simulink model "sldemo_househeatsolution"  (R2026a)
settings: Solver=ode45  StopTime=172800  FixedStep=1  AbsTol=1e-6
model workspace (MATLAB code in the model file):
  | % load initial conditions and physical properties from file
  | 
  | sldemo_househeat_data
undefined symbols (not defined in the file): c, cost, M, Mdot, Req, THeater, TinIC
libraries: simulink_extras x3
Description:
  | Thermal Model of a House
  | 
  | This demo illustrates how you can use Simulink(R) to create the thermal model of
  | a house. This system models the outdoor environment, the thermal
  | characteristics of the house, and the house heating system.
  | 
  | The sldemo_househeat_data.m file initializes data in the model workspace.
  | To make changes, you can edit the model workspace directly or edit the MATLAB(R) file
  | and re-load the model workspace.
  | 
  | To view the model workspace, select View > Model Explorer
  | from the Simulink editor.
  | 
  | Note: Time is given in units of hours
settings Model: ExtModeTrigMode=oneshot  ExtModeArmWhenConnect=off  ExtModeAutoUpdateStatusClock=off  Creator=The MathWorks, Inc.  LastModifiedBy=The MathWorks, Inc.
settings DataIOCC: ExternalInput=[]  InitialState=[]
settings OptimizationCC: BooleanDataType=off  InitFltsAndDblsToZero=on  BufferReusableBoundary=off
settings DebuggingCC: SaveWithParameterizedLinksMsg=none  UnderspecifiedInitializationDetection=Classic  SignalResolutionControl=TryResolveAllWithWarning  MultiTaskDSMMsg=warning  MultiTaskCondExecSysMsg=none  IntegerOverflowMsg=none  BusObjectLabelMismatch=none  IntegerSaturationMsg=none
settings HardwareCC: ProdHWDeviceType=32-bit Generic  TargetUnknown=on
settings GRTTargetCC: TargetFcnLib=ansi_tfl_tmw.mat  CombineOutputUpdateFcns=off  GRTInterface=on

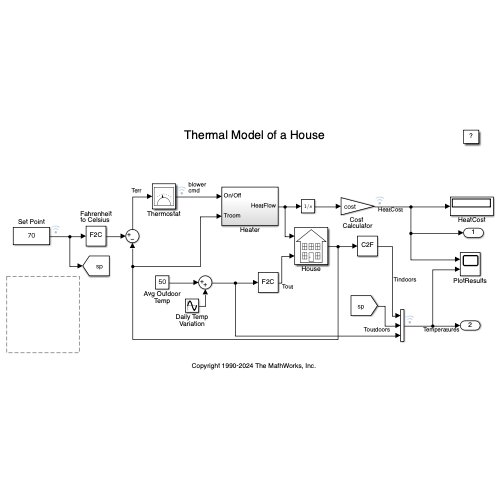
[thumbnail: Simulink's stored preview of the top-level diagram]
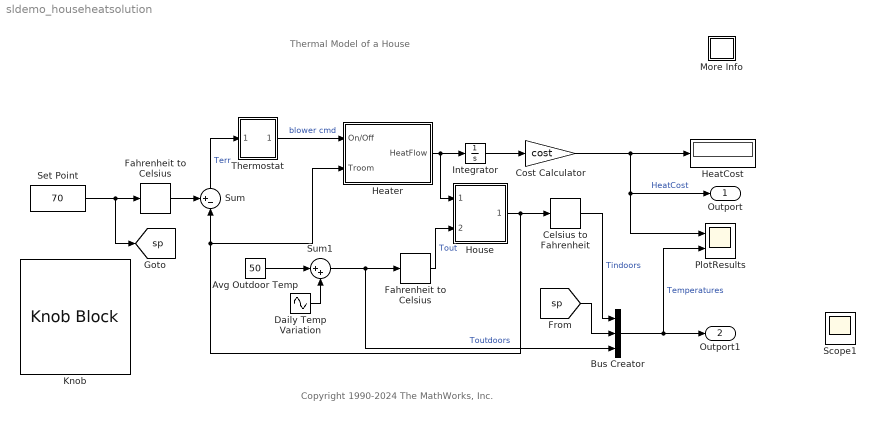
== system sldemo_househeatsolution ==
  note: Thermal Model of a House
  note: Copyright 1990-2024 The MathWorks, Inc.
  Avg Outdoor Temp : Constant  Value=50
  Bus Creator : BusCreator  Inputs=3
  Celsius to Fahrenheit : simulink_extras/Transformations/Celsius to Fahrenheit
  Cost Calculator : Gain  Gain=cost  SaturateOnIntegerOverflow=on  OutDataTypeStr=Inherit: Same as input  ParamDataTypeStr=Inherit: Same as input
  Daily Temp Variation : Sin  Amplitude=15  Frequency=(2*pi)/(24*3600)  SampleTime=0
  Fahrenheit to Celsius : simulink_extras/Transformations/Fahrenheit to Celsius
  "Fahrenheit to Celsius " : simulink_extras/Transformations/Fahrenheit to Celsius
  HeatCost : Display
  Heater : Subsystem
  House : Subsystem
      mask Display: image('HouseHeatHousePix.svg')
  Integrator : Integrator
  Knob : KnobBlock  ScaleMin=60
  More Info : Subsystem
      settings: OpenFcn=showExample('simulink_general/sldemo_househeatExample')
      mask Display: disp('?')
  PlotResults : Scope  NumInputPorts=2
      settings: ActiveDisplayYMinimum=-3  ActiveDisplayYMaximum=37  YLabel=HeatCost (in $)
  Set Point : Constant  Value=70
  Sum : Sum  Inputs=+-|  InputSameDT=on  SaturateOnIntegerOverflow=on  OutDataTypeStr=Inherit: Same as first input
  Sum1 : Sum  Inputs=|++  InputSameDT=on  SaturateOnIntegerOverflow=on  OutDataTypeStr=Inherit: Same as first input
  Thermostat : Subsystem
      mask Display: image('HouseHeatThermostatPix.svg')
  Outport : Outport
  Outport1 : Outport  Port=2
  Scope1 : Scope
      settings: ActiveDisplayYMinimum=-0.125  ActiveDisplayYMaximum=1.125
  tag scope: sp=global
  wires:
  Integrator/1 -> Cost Calculator/1
  Thermostat/1(Blower switch) -> Heater/1(On/Off)  "blower cmd"
  Sum/1 -> Thermostat/1(Terr)  "Terr"
  House/1(Room Temp Troom) -> Celsius to Fahrenheit/1, Heater/2(Troom), Sum/2
  Daily Temp Variation/1 -> Sum1/2
  Sum1/1 -> Fahrenheit to Celsius/1, Bus Creator/3  "Toutdoors"
  Avg Outdoor Temp/1 -> Sum1/1
  Celsius to Fahrenheit/1 -> Bus Creator/1  "Tindoors"
  Fahrenheit to Celsius/1 -> House/2(Outdoor Temp Tout)  "Tout"
  Heater/1(HeatFlow) -> Integrator/1, House/1(Heater QDot In)
  Bus Creator/1 -> Outport1/1, PlotResults/2  "Temperatures"
  Cost Calculator/1 -> Outport/1, PlotResults/1, HeatCost/1  "HeatCost"
  "Fahrenheit to Celsius "/1 -> Sum/1
  Set Point/1 -> [sp], "Fahrenheit to Celsius "/1
  [sp] -> Bus Creator/2

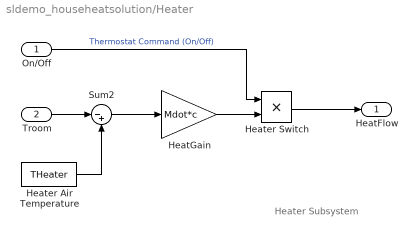
== system sldemo_househeatsolution/Heater ==
  note: Heater Subsystem
  On/Off : Inport
  Troom : Inport  Port=2
  HeatGain : Gain  Gain=Mdot*c
  Heater Air Temperature : Constant  Value=THeater
  Heater Switch : Product  RndMeth=Zero
  Sum2 : Sum  Inputs=|-+
  HeatFlow : Outport  VectorParamsAs1DForOutWhenUnconnected=off
  wires:
  Heater Air Temperature/1 -> Sum2/2
  Troom/1 -> Sum2/1
  Sum2/1 -> HeatGain/1
  On/Off/1 -> Heater Switch/1  "Thermostat Command (On/Off)"
  HeatGain/1 -> Heater Switch/2
  Heater Switch/1 -> HeatFlow/1

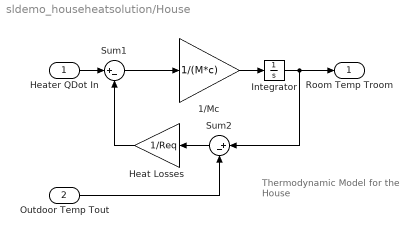
== system sldemo_househeatsolution/House ==
  note: Thermodynamic Model
      | for the House
  Heater QDot In : Inport
  Outdoor Temp Tout : Inport  Port=2
  1/Mc : Gain  Gain=1/(M*c)  SaturateOnIntegerOverflow=on  OutDataTypeStr=Inherit: Same as input  ParamDataTypeStr=Inherit: Same as input
  Heat Losses : Gain  Gain=1/Req  SaturateOnIntegerOverflow=on  OutDataTypeStr=Inherit: Same as input  ParamDataTypeStr=Inherit: Same as input
  Integrator : Integrator  InitialCondition=TinIC
  Sum1 : Sum  Inputs=|+-  InputSameDT=on  SaturateOnIntegerOverflow=on  OutDataTypeStr=Inherit: Same as first input
  Sum2 : Sum  Inputs=|+-  InputSameDT=on  SaturateOnIntegerOverflow=on  OutDataTypeStr=Inherit: Same as first input
  Room Temp Troom : Outport  InitialOutput=0  VectorParamsAs1DForOutWhenUnconnected=off
  wires:
  Outdoor Temp Tout/1 -> Sum2/2
  Heater QDot In/1 -> Sum1/1
  Sum1/1 -> 1/Mc/1
  Sum2/1 -> Heat Losses/1
  Heat Losses/1 -> Sum1/2
  1/Mc/1 -> Integrator/1
  Integrator/1 -> Sum2/1, Room Temp Troom/1

== system sldemo_househeatsolution/More Info ==

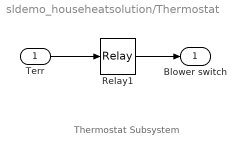
== system sldemo_househeatsolution/Thermostat ==
  note: Thermostat Subsystem
  Terr : Inport
  Relay1 : Relay  OnSwitchValue=5*(5/9)  OffSwitchValue=-5*(5/9)
  Blower switch : Outport  InitialOutput=0  VectorParamsAs1DForOutWhenUnconnected=off
  wires:
  Terr/1 -> Relay1/1
  Relay1/1 -> Blower switch/1
